simulink model "car"  (R2017b)
settings: Solver=VariableStepAuto  StartTime=0.0  StopTime=100.0  RelTol=1e-3
libraries: fuzblock x1
settings Model: Creator=kian  LastModifiedBy=kian

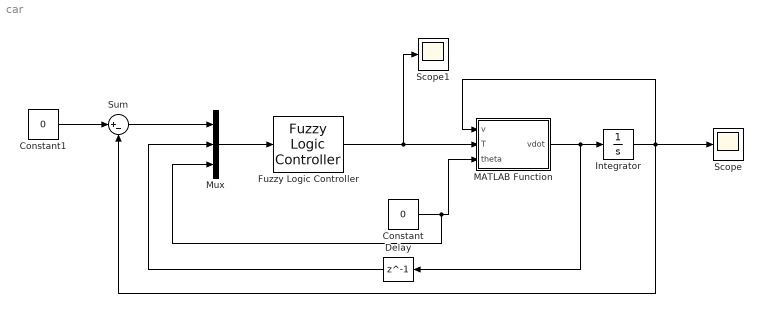
== system car ==
  Constant : Constant  Value=0
  Constant1 : Constant  Value=0
  Delay : Delay  DelayLength=1
  Fuzzy Logic Controller : fuzblock/Fuzzy Logic  Controller  FIS='test.fis'  OutputSampleNumber=101  DataType=double  FuzzifiedInputs=off  RuleFiringStrengths=off  RuleOutputs=off  AggregatedOutputs=off  SimulateUsing=Interpreted execution
  Integrator : Integrator
  MATLAB Function : MATLAB Function  TreatAsAtomicUnit=on
  Mux : Mux  Inputs=3
  Scope : Scope
  Scope1 : Scope
  Sum : Sum  Inputs=|+-
  wires:
  MATLAB Function/1(vdot) -> Delay/1, Integrator/1
  Constant/1 -> Mux/3, MATLAB Function/3(theta)
  Mux/1 -> Fuzzy Logic Controller/1
  Constant1/1 -> Sum/1
  Sum/1 -> Mux/1
  Integrator/1 -> MATLAB Function/1(v), Scope/1, Sum/2
  Delay/1 -> Mux/2
  Fuzzy Logic Controller/1 -> MATLAB Function/2(T), Scope1/1

== matlab function car/MATLAB Function ==
  data: v input; vdot output; T input; theta input
function vdot = car(v, T, theta)
    vdot = -0.1*v + [-1 0.1]*transpose([-T theta]);
end
